simulink model "Uniform_motion"  (R2022a)
settings: Solver=VariableStepAuto  StartTime=0.0  StopTime=10.0  RelTol=1e-3
model workspace (MAT data in the model file):
  ratio1 = 6.09
  ratio2 = 3.09
  ratio3 = 1.71
  ratio4 = 1
undefined symbols (not defined in the file): f, g, i0, kt, m2, r
libraries: simulink x1
settings Model: DataDictionary=Vehicle_paramiter.sldd  Creator=cht  LastModifiedBy=cht
settings DataIOCC: SaveFormat=Array  SaveOutput=off  InspectSignalLogs=on  SaveTime=off  ReturnWorkspaceOutputs=off

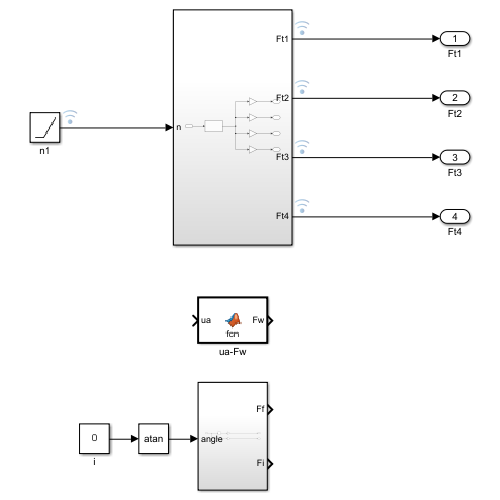
[thumbnail: Simulink's stored preview of the top-level diagram]
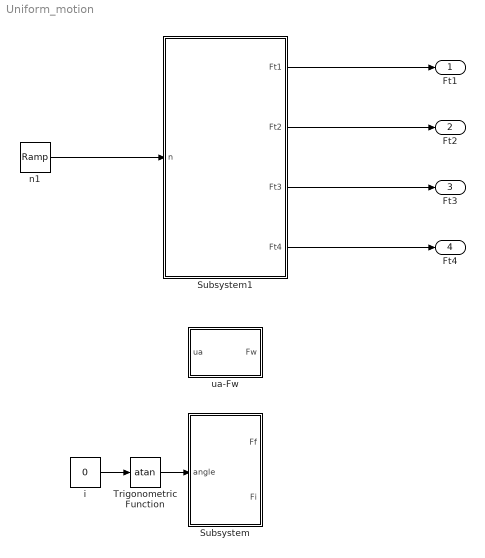
== system Uniform_motion ==
  Subsystem : Subsystem
  Subsystem1 : Subsystem
  Trigonometric Function : Trigonometry  Operator=atan
  i : Constant  Value=0
  n1 : simulink/Sources/Ramp  slope=340  start=0  InitialOutput=600
  ua-Fw : MATLAB Function  TreatAsAtomicUnit=on
  Ft1 : Outport
  Ft2 : Outport  Port=2
  Ft3 : Outport  Port=3
  Ft4 : Outport  Port=4
  wires:
  Trigonometric Function/1 -> Subsystem/1(angle)
  i/1 -> Trigonometric Function/1
  Subsystem1/1(Ft1) -> Ft1/1
  Subsystem1/2(Ft2) -> Ft2/1
  Subsystem1/3(Ft3) -> Ft3/1
  Subsystem1/4(Ft4) -> Ft4/1
  n1/1 -> Subsystem1/1(n)

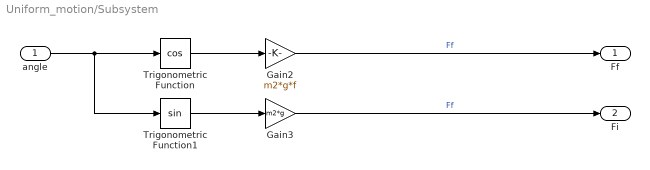
== system Uniform_motion/Subsystem ==
  angle : Inport
  Gain2 : Gain  Gain=m2*g*f
  Gain3 : Gain  Gain=m2*g
  Trigonometric Function : Trigonometry  Operator=cos
  Trigonometric Function1 : Trigonometry
  Ff : Outport
  Fi : Outport  Port=2
  wires:
  Gain3/1 -> Fi/1  "Ff"
  angle/1 -> Trigonometric Function1/1, Trigonometric Function/1
  Trigonometric Function1/1 -> Gain3/1
  Trigonometric Function/1 -> Gain2/1
  Gain2/1 -> Ff/1  "Ff"

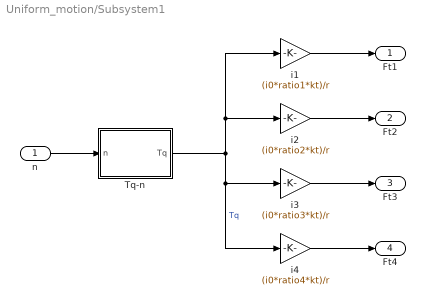
== system Uniform_motion/Subsystem1 ==
  n : Inport
  Tq-n : MATLAB Function  TreatAsAtomicUnit=on
  i1 : Gain  Gain=(i0*ratio1*kt)/r
  i2 : Gain  Gain=(i0*ratio2*kt)/r
  i3 : Gain  Gain=(i0*ratio3*kt)/r
  i4 : Gain  Gain=(i0*ratio4*kt)/r
  Ft1 : Outport
  Ft2 : Outport  Port=2
  Ft3 : Outport  Port=3
  Ft4 : Outport  Port=4
  wires:
  Tq-n/1(Tq) -> i4/1, i3/1, i1/1, i2/1  "Tq"
  n/1 -> Tq-n/1(n)
  i2/1 -> Ft2/1
  i1/1 -> Ft1/1
  i3/1 -> Ft3/1
  i4/1 -> Ft4/1

== matlab function Uniform_motion/Subsystem1/Tq-n ==
  data: n input; Tq output
function Tq = fcn(n)
%#codegen

Tq = -19.313+295.27*(n/1000)-165.44*(n/1000)^2+40.874*(n/1000)^3-3.8445*(n/1000)^4;

== matlab function Uniform_motion/ua-Fw ==
  data: ua input; Fw output
function Fw = fcn(ua)
%#codegen
CA=2.77;
Fw =(CA*ua*ua)/21.15;
